simulink model "P1_1a_solution"  (R2021b)
settings: Solver=VariableStepAuto  StartTime=0.0  StopTime=10.0  RelTol=1e-3
undefined symbols (not defined in the file or in its folder): a3, g, L, x0, y0, z0
settings Model: Creator=Sebastián  LastModifiedBy=Sebastián

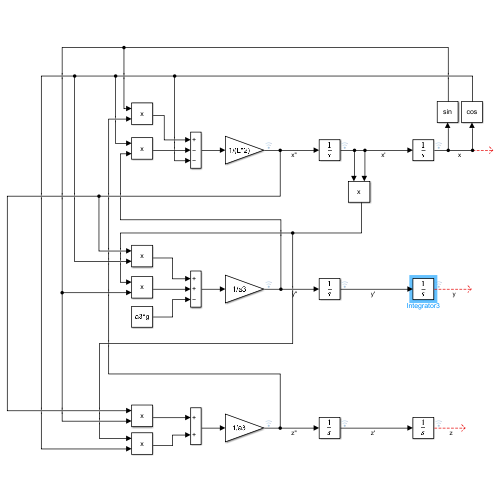
[thumbnail: Simulink's stored preview of the top-level diagram]
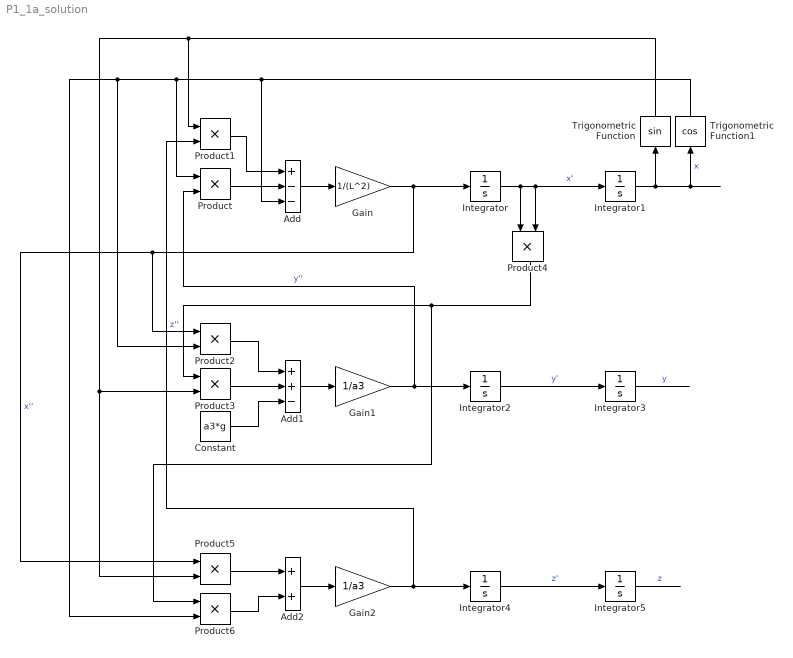
== system P1_1a_solution ==
  Add : Sum  Inputs=+--
  Add1 : Sum  Inputs=++-
  Add2 : Sum
  Constant : Constant  Value=a3*g
  Gain : Gain  Gain=1/(L^2)
  Gain1 : Gain  Gain=1/a3
  Gain2 : Gain  Gain=1/a3
  Integrator : Integrator  InitialCondition=x0(2)
  Integrator1 : Integrator  InitialCondition=x0(1)
  Integrator2 : Integrator  InitialCondition=y0(2)
  Integrator3 : Integrator  InitialCondition=y0(1)
  Integrator4 : Integrator  InitialCondition=z0(2)
  Integrator5 : Integrator  InitialCondition=z0(1)
  Product{,1..6} (7 alike) : Product
  Trigonometric Function : Trigonometry
  Trigonometric Function1 : Trigonometry  Operator=cos
  wires:
  Gain/1 -> Product2/1, Product5/1, Integrator/1  "x''"
  Integrator/1 -> Integrator1/1, Product4/2, Product4/1  "x'"
  Add/1 -> Gain/1
  Integrator2/1 -> Integrator3/1  "y'"
  Gain1/1 -> Product/2, Integrator2/1  "y''"
  Add1/1 -> Gain1/1
  Integrator4/1 -> Integrator5/1  "z'"
  Gain2/1 -> Product1/2, Integrator4/1  "z''"
  Add2/1 -> Gain2/1
  Integrator1/1 -> Trigonometric Function/1, Trigonometric Function1/1  "x"
  Trigonometric Function1/1 -> Add/3, Product/1, Product6/2, Product2/2
  Product/1 -> Add/2
  Product1/1 -> Add/1
  Trigonometric Function/1 -> Product1/1, Product5/2, Product3/2
  Constant/1 -> Add1/3
  Product3/1 -> Add1/2
  Product2/1 -> Add1/1
  Product4/1 -> Product6/1, Product3/1
  Integrator3/1 -> ?  "y"
  Product5/1 -> Add2/1
  Product6/1 -> Add2/2
  Integrator5/1 -> ?  "z"
